simulink library "ddm"  (R2021b)
settings: Solver=VariableStepAuto  StartTime=0.0  StopTime=10.0  RelTol=1e-3
undefined symbols (not defined in the file or in its folder): ENUM_ADASACCSTA_ERROR, ENUM_ADASACCSTA_OFF, ENUM_ADASACCSTA_STANDBY, ENUM_ADASISASTA_OFF, ENUM_ALLOWMOV_ALLOWREADY, ENUM_APS, ENUM_BRKSTA_ERROR, ENUM_BRKSTA_OFF, ENUM_BRKSTA_ON, ENUM_BRKSW_INVALID, ENUM_BRKSW_OFF, ENUM_BRKSW_ON, ENUM_CHGPREACTERRSTA_OBCPRE, ENUM_DCDCFAULTSTA_ANYFAULTLV1, ENUM_DCDCFAULTSTA_ANYFAULTLV2, ENUM_DRIVETRAIN_AWD, ENUM_DRIVETRAIN_FWD, ENUM_DRIVETRAIN_RWD, ENUM_DRSEATSTA_INVALID, ENUM_EDUDRTSTA_NORMAL, ENUM_EPBSTA_APPLIED, ENUM_EPBSTA_RELEASED, ENUM_HVBATTREADYPRE_READY, ENUM_MCUWARN_LV0, ENUM_MCUWARN_LV1, ENUM_MCUWARN_LV2, ENUM_MCUWARN_LV3, ENUM_MCUWARN_NOERROR, ENUM_OBCFAULTSTA_ANYFAULT, ENUM_PAS_R2F2, ENUM_PDFAULT_BATTPDFAIL, ENUM_PDFAULT_DCDCDISABLE, ENUM_PDFAULT_MCUDISABLE, ENUM_PDFAULT_MCUDISCHRG, ENUM_POWERSTA_OFF, ENUM_POWERSTA_ON, ENUM_POWERSTA_READY, ENUM_POWERSTA_STANDBY, ENUM_PRESSINDI_LOW, ENUM_PUFAULT_BATTUPFAIL, ENUM_PUFAULT_DCDCENABLEFAIL, ENUM_PUFAULT_PRECHRGCHKFAIL, ENUM_PUFAULT_SAFETYCHKFAIL, ENUM_PUSTATE_COMPLETED, ENUM_PWRSTASW_OFF, ENUM_PWRSTASW_OFFA, ENUM_PWRSTASW_OFFCHVCHRG, ENUM_PWRSTASW_OFFCLVCHRG, ENUM_PWRSTASW_ON, ENUM_PWRSTASW_ONHVCHRG, ENUM_PWRSTASW_READY, ENUM_PWRSTASW_STANDBY, ENUM_RANGESTA_12IN, ENUM_SHIFTCOMMAND_D, ENUM_SHIFTCOMMAND_N, ENUM_SHIFTCOMMAND_P, ENUM_SHIFTCOMMAND_R, ENUM_VEHMALFUNLV_2ND, ENUM_VEHMALFUNLV_3RD, ENUM_VEHMALFUNLV_4TH ... (+835)
libraries: hcu_lib x750, $bdroot x12, simulink x5
(part 6 of 28)

== system ddm/DDM/DDM/APM/Subsystem8 ==
  USSSta_flg : Inport
  VPMM_SysPwrSta_enum : Inport  Port=2
  VAPM_SNSRLayout_enum : Inport  Port=3
  Constant1 : Constant  Value=ENUM_PWRSTASW_READY
  Constant17 : Constant  Value=ENUM_PWRSTASW_READY
  Constant2 : Constant  Value=ENUM_PWRSTASW_ON
  Constant25 : Constant  Value=FALSE
  Constant3 : Constant  Value=ENUM_PWRSTASW_ON
  Constant5 : Constant  Value=ENUM_APS
  Equal{1..3,5..6} (5 alike) : RelationalOperator  Operator===  OutDataTypeStr=boolean  RndMeth=Simplest
  Logical Operator1 : Logic  Operator=NOT  AllPortsSameDT=off  OutDataTypeStr=boolean
  Logical Operator13 : Logic  Operator=OR  AllPortsSameDT=off  OutDataTypeStr=boolean
  Logical Operator2 : Logic  AllPortsSameDT=off  OutDataTypeStr=boolean
  Logical Operator3 : Logic  Operator=OR  AllPortsSameDT=off  OutDataTypeStr=boolean
  Logical Operator4 : Logic  AllPortsSameDT=off  OutDataTypeStr=boolean
  Switch2 : Switch  Criteria=u2 ~= 0
  Pass_flg : Outport
  CFS_flg : Outport  Port=2
  wires:
  [VPMM_SysPwrSta_enum] -> Equal2/1
  Equal6/1 -> Logical Operator13/1
  Constant17/1 -> Equal2/2
  Constant3/1 -> Equal6/2
  Equal2/1 -> Logical Operator13/2
  [VPMM_SysPwrSta_enum] -> Equal6/1
  Logical Operator13/1 -> Logical Operator2/1
  Logical Operator1/1 -> Logical Operator2/2
  Logical Operator2/1 -> Pass_flg/1
  Logical Operator3/1 -> Logical Operator4/2
  [VPMM_SysPwrSta_enum] -> Equal3/1
  Equal1/1 -> Logical Operator3/2
  Constant2/1 -> Equal3/2
  Constant1/1 -> Equal1/2
  Equal3/1 -> Logical Operator3/1
  [VPMM_SysPwrSta_enum] -> Equal1/1
  Switch2/1 -> Logical Operator4/1, Logical Operator1/1
  Logical Operator4/1 -> CFS_flg/1
  VPMM_SysPwrSta_enum/1 -> [VPMM_SysPwrSta_enum]
  Constant5/1 -> Equal5/2
  VAPM_SNSRLayout_enum/1 -> Equal5/1
  Equal5/1 -> Switch2/2
  Constant25/1 -> Switch2/3
  USSSta_flg/1 -> Switch2/1

== system ddm/DDM/DDM/APM/Subsystem9 ==
  USSSta_flg : Inport
  VPMM_SysPwrSta_enum : Inport  Port=2
  VAPM_SNSRLayout_enum : Inport  Port=3
  Constant1 : Constant  Value=ENUM_PWRSTASW_READY
  Constant17 : Constant  Value=ENUM_PWRSTASW_READY
  Constant2 : Constant  Value=ENUM_PWRSTASW_ON
  Constant25 : Constant  Value=FALSE
  Constant3 : Constant  Value=ENUM_PWRSTASW_ON
  Constant5 : Constant  Value=ENUM_APS
  Equal{1..3,5..6} (5 alike) : RelationalOperator  Operator===  OutDataTypeStr=boolean  RndMeth=Simplest
  Logical Operator1 : Logic  Operator=NOT  AllPortsSameDT=off  OutDataTypeStr=boolean
  Logical Operator13 : Logic  Operator=OR  AllPortsSameDT=off  OutDataTypeStr=boolean
  Logical Operator2 : Logic  AllPortsSameDT=off  OutDataTypeStr=boolean
  Logical Operator3 : Logic  Operator=OR  AllPortsSameDT=off  OutDataTypeStr=boolean
  Logical Operator4 : Logic  AllPortsSameDT=off  OutDataTypeStr=boolean
  Switch2 : Switch  Criteria=u2 ~= 0
  Pass_flg : Outport
  CFS_flg : Outport  Port=2
  wires:
  [VPMM_SysPwrSta_enum] -> Equal2/1
  Equal6/1 -> Logical Operator13/1
  Constant17/1 -> Equal2/2
  Constant3/1 -> Equal6/2
  Equal2/1 -> Logical Operator13/2
  [VPMM_SysPwrSta_enum] -> Equal6/1
  Logical Operator13/1 -> Logical Operator2/1
  Logical Operator1/1 -> Logical Operator2/2
  Logical Operator2/1 -> Pass_flg/1
  Logical Operator3/1 -> Logical Operator4/2
  [VPMM_SysPwrSta_enum] -> Equal3/1
  Equal1/1 -> Logical Operator3/2
  Constant2/1 -> Equal3/2
  Constant1/1 -> Equal1/2
  Equal3/1 -> Logical Operator3/1
  [VPMM_SysPwrSta_enum] -> Equal1/1
  Switch2/1 -> Logical Operator4/1, Logical Operator1/1
  Logical Operator4/1 -> CFS_flg/1
  VPMM_SysPwrSta_enum/1 -> [VPMM_SysPwrSta_enum]
  Constant5/1 -> Equal5/2
  VAPM_SNSRLayout_enum/1 -> Equal5/1
  Equal5/1 -> Switch2/2
  Constant25/1 -> Switch2/3
  USSSta_flg/1 -> Switch2/1

== system ddm/DDM/DDM/PMM/Brake switch signal abnormal ==
  task_time_s : Inport
  VPMM_PwrStaSW_enum : Inport  Port=2
  VPMM_PowerSta_enum : Inport  Port=3
  VINP_BrakeSWGPIO_flg : Inport  Port=4
  VINP_BrakeLampSW_flg : Inport  Port=5
  VDDM_ESC5NoComCFS_flg : Inport  Port=6
  VDDM_ESC5RCErrCFS_flg : Inport  Port=7
  VDDM_ESC5CSErrCFS_flg : Inport  Port=8
  VINP_DrStdAErrSta_enum : Inport  Port=9
  VINP_BrkSWSta_flg : Inport  Port=10
  VDDM_ESC7NoComCFS_flg : Inport  Port=11
  VDDM_ESC7RCErrCFS_flg : Inport  Port=12
  VDDM_ESC7CSErrCFS_flg : Inport  Port=13
  VINP_BrkPedalPosSta_enum : Inport  Port=14
  VINP_BrkPedalPos_pct : Inport  Port=15
  DTC_clear_request : Inport  Port=16
  Brake switch signal abnormal : Subsystem
  Brake switch signal abnormal and no backup signal : Subsystem
  Constant : Constant  Value=TRUE
  Constant1 : Constant  Value=ENUM_BRKSTA_ERROR
  Constant2 : Constant  Value=ENUM_BRKSTA_ON
  Constant3 : Constant  Value=ENUM_BRKSTA_OFF
  Constant4 : Constant  Value=FALSE
  Constant5 : Constant  Value=ENUM_BRKSTA_ERROR
  Constant6 : Constant  Value=ENUM_BRKSTA_ON
  Constant7 : Constant  Value=ENUM_BRKSTA_OFF
  Constant8 : Constant  Value=KDDM_BrkPedalPos_pct
  Equal : RelationalOperator  Operator===  OutDataTypeStr=boolean  RndMeth=Simplest
  Equal1 : RelationalOperator  Operator===  OutDataTypeStr=boolean  RndMeth=Simplest
  Equal2 : RelationalOperator  OutDataTypeStr=boolean  RndMeth=Simplest
  Logical Operator : Logic  Operator=OR  Inputs=4  AllPortsSameDT=off  OutDataTypeStr=boolean
  Logical Operator1 : Logic  Operator=OR  Inputs=4  AllPortsSameDT=off  OutDataTypeStr=boolean
  Subsystem : Subsystem
  Switch{,1..3} (4 alike) : Switch  Criteria=u2 > Threshold
  VDDM_BrkSWErrDTC_raw32 : Outport
  VDDM_BrkSWNoBacDTC_raw32 : Outport  Port=2
  VDDM_BrakeSW_enum : Outport  Port=3
  VDDM_CANBrkSW2Sta_enum : Outport  Port=4
  VDDM_BrkPedalPosSta_enum : Outport  Port=5
  VDDM_EDriveSysErrBrake_flg : Outport  Port=6
  VDDM_VCUBrkSWSta_enum : Outport  Port=7
  wires:
  [VDDM_BrakeSW_enum] -> Brake switch signal abnormal and no backup signal/7(VDDM_BrakeSW_enum)
  [VDDM_BrkSWPass_flg] -> Brake switch signal abnormal and no backup signal/5(BrkSWPass)
  [VDDM_BrkSWNoBac_flg] -> Brake switch signal abnormal and no backup signal/4(BrkSWNoBac)
  [VDDM_BrkSWPass_flg] -> Brake switch signal abnormal/5(BrkSWPass)
  [VDDM_BrkSWErr_flg] -> Brake switch signal abnormal/4(BrkSWErr)
  Subsystem/3(BrkSWPass) -> [VDDM_BrkSWPass_flg]  "VDDM_BrkSWPass_flg"
  Subsystem/2(BrkSWNoBac) -> [VDDM_BrkSWNoBac_flg]  "VDDM_BrkSWNoBac_flg"
  Subsystem/4(VDDM_BrakeSW_enum) -> [VDDM_BrakeSW_enum]  "VDDM_BrakeSW_enum"
  Subsystem/1(BrkSWErr) -> [VDDM_BrkSWErr_flg]  "VDDM_BrkSWErr_flg"
  VINP_BrakeLampSW_flg/1 -> Subsystem/3(Brake_Stop_Lamp)
  VINP_BrakeSWGPIO_flg/1 -> Subsystem/2(BrakeSW)
  [VDDM_BrkPedalPosSta_enum] -> Subsystem/4(BrkPedalPos_enum)
  [VDDM_CANBrkSW2Sta_enum] -> Subsystem/1(VDDM_CANBSW2S_enum)
  [DTC_clear_request] -> Brake switch signal abnormal and no backup signal/6(DTC_clear_request)
  [DTC_clear_request] -> Brake switch signal abnormal/6(DTC_clear_request)
  DTC_clear_request/1 -> [DTC_clear_request]
  Brake switch signal abnormal and no backup signal/2(VDDM_VCUBrkSWSta_enum) -> VDDM_VCUBrkSWSta_enum/1
  Brake switch signal abnormal/2(VDDM_EDriveSysErrBrake_flg) -> VDDM_EDriveSysErrBrake_flg/1
  [VDDM_BrakeSW_enum] -> VDDM_BrakeSW_enum/1
  [VDDM_CANBrkSW2Sta_enum] -> VDDM_CANBrkSW2Sta_enum/1
  [VDDM_BrkPedalPosSta_enum] -> VDDM_BrkPedalPosSta_enum/1
  Switch2/1 -> [VDDM_BrkPedalPosSta_enum]  "VDDM_BrkPedalPosSta_enum"
  Switch/1 -> [VDDM_CANBrkSW2Sta_enum]  "VDDM_CANBrkSW2Sta_enum"
  Brake switch signal abnormal and no backup signal/1(VDDM_BrkSWNoBacDTC_raw32) -> VDDM_BrkSWNoBacDTC_raw32/1
  Brake switch signal abnormal/1(VDDM_BrkSWErrDTC_raw32) -> VDDM_BrkSWErrDTC_raw32/1
  Equal2/1 -> Switch3/2
  Constant8/1 -> Equal2/2
  VINP_BrkPedalPos_pct/1 -> Equal2/1
  VINP_BrkPedalPosSta_enum/1 -> Equal1/1
  Constant4/1 -> Equal1/2
  VDDM_ESC7CSErrCFS_flg/1 -> Logical Operator1/3
  VDDM_ESC7RCErrCFS_flg/1 -> Logical Operator1/2
  VDDM_ESC7NoComCFS_flg/1 -> Logical Operator1/1
  Equal1/1 -> Logical Operator1/4
  Switch3/1 -> Switch2/3
  Logical Operator1/1 -> Switch2/2
  Constant5/1 -> Switch2/1
  Constant6/1 -> Switch3/1
  Constant7/1 -> Switch3/3
  Constant3/1 -> Switch1/3
  Constant2/1 -> Switch1/1
  VINP_BrkSWSta_flg/1 -> Switch1/2
  Constant1/1 -> Switch/1
  Logical Operator/1 -> Switch/2
  Switch1/1 -> Switch/3
  Equal/1 -> Logical Operator/4
  VDDM_ESC5NoComCFS_flg/1 -> Logical Operator/1
  VDDM_ESC5RCErrCFS_flg/1 -> Logical Operator/2
  VDDM_ESC5CSErrCFS_flg/1 -> Logical Operator/3
  Constant/1 -> Equal/2
  VINP_DrStdAErrSta_enum/1 -> Equal/1
  task_time_s/1 -> [task_time_s]
  VPMM_PwrStaSW_enum/1 -> [VPMM_PwrStaSW_enum]
  VPMM_PowerSta_enum/1 -> [VPMM_PowerSta_enum]
  [task_time_s] -> Brake switch signal abnormal/1(task_time_s)
  [VPMM_PwrStaSW_enum] -> Brake switch signal abnormal/3(VPMM_PwrStaSW_enum)
  [VPMM_PowerSta_enum] -> Brake switch signal abnormal/2(VPMM_PowerSta_enum)
  [task_time_s] -> Brake switch signal abnormal and no backup signal/1(task_time_s)
  [VPMM_PowerSta_enum] -> Brake switch signal abnormal and no backup signal/2(VPMM_PowerSta_enum)
  [VPMM_PwrStaSW_enum] -> Brake switch signal abnormal and no backup signal/3(VPMM_PwrStaSW_enum)

== system ddm/DDM/DDM/PMM/Comm err ==
  note: CAN1 EPAS2
  note: CAN3 BMS6
  note: CAN3 BMS1
  note: CAN3 CCU1
  note: CAN3 CCU2
  note: CAN1 ABM1
  task_time_s : Inport
  VPMM_PowerSta_enum : Inport  Port=2
  VPMM_PwrStaSW_enum : Inport  Port=3
  VDDM_C3BMS6RCChk_flg : Inport  Port=4
  VDDM_C3BMS6CSChk_flg : Inport  Port=5
  VDDM_C3BMS6LCChk_flg : Inport  Port=6
  VDDM_C3BMS1RCChk_flg : Inport  Port=7
  VDDM_C3BMS1CSChk_flg : Inport  Port=8
  VDDM_C3BMS1LCChk_flg : Inport  Port=9
  VDDM_C3CCU1RCChk_flg : Inport  Port=10
  VDDM_C3CCU1CSChk_flg : Inport  Port=11
  VDDM_C3CCU1LCChk_flg : Inport  Port=12
  VDDM_C3CCU2RCChk_flg : Inport  Port=13
  VDDM_C3CCU2CSChk_flg : Inport  Port=14
  VDDM_C3CCU2LCChk_flg : Inport  Port=15
  VDDM_C1ABM1RCChk_flg : Inport  Port=16
  VDDM_C1ABM1CSChk_flg : Inport  Port=17
  VDDM_C1ABM1LCChk_flg : Inport  Port=18
  No_CAN3_BUS_OFF : Inport  Port=19
  No_CAN1_BUS_OFF : Inport  Port=20
  DTC_clear_request : Inport  Port=21
  VDDM_C1EPAS2LCChk_flg : Inport  Port=22
  FDC lost communication with EPAS2 : Subsystem
  OR : Logic  Operator=OR  Inputs=3  AllPortsSameDT=off  OutDataTypeStr=boolean
  The CAN signal between VCU and ABM1 is discontinuous : Subsystem
  The CAN signal between VCU and ABM1 is incomplete : Subsystem
  The CAN signal between VCU and BMS1 is discontinuous : Subsystem
  The CAN signal between VCU and BMS1 is incomplete : Subsystem
  The CAN signal between VCU and BMS6 is discontinuous : Subsystem
  The CAN signal between VCU and BMS6 is incomplete : Subsystem
  The CAN signal between VCU and CCU1 is discontinuous : Subsystem
  The CAN signal between VCU and CCU1 is incomplete : Subsystem
  The CAN signal between VCU and CCU2 is discontinuous : Subsystem
  The CAN signal between VCU and CCU2 is incomplete : Subsystem
  VCU lost communication with ABM1 : Subsystem
  VCU lost communication with BMS1 : Subsystem
  VCU lost communication with BMS6 : Subsystem
  VCU lost communication with CCU1 : Subsystem
  VCU lost communication with CCU2 : Subsystem
  VDDM_C3BMS6RCDTC_raw32 : Outport
  VDDM_C3BMS6CSDTC_raw32 : Outport  Port=2
  VDDM_C3BMS6LCDTC_raw32 : Outport  Port=3
  VDDM_C3BMS1RCDTC_raw32 : Outport  Port=4
  VDDM_C3BMS1CSDTC_raw32 : Outport  Port=5
  VDDM_C3BMS1LCDTC_raw32 : Outport  Port=6
  VDDM_C3CCU1RCDTC_raw32 : Outport  Port=7
  VDDM_C3CCU1CSDTC_raw32 : Outport  Port=8
  VDDM_C3CCU1LCDTC_raw32 : Outport  Port=9
  VDDM_C3CCU2RCDTC_raw32 : Outport  Port=10
  VDDM_C3CCU2CSDTC_raw32 : Outport  Port=11
  VDDM_C3CCU2LCDTC_raw32 : Outport  Port=12
  VDDM_C1ABM1RCDTC_raw32 : Outport  Port=13
  VDDM_C1ABM1CSDTC_raw32 : Outport  Port=14
  VDDM_C1ABM1LCDTC_raw32 : Outport  Port=15
  VDDM_EDriveSysErrABMCAN_flg : Outport  Port=16
  VDDM_C3BMS6CSCFS_flg : Outport  Port=17
  VDDM_C3BMS6RCCFS_flg : Outport  Port=18
  VDDM_C3BMS6LCCFS_flg : Outport  Port=19
  VDDM_C3CCU2CSCFS_flg : Outport  Port=20
  VDDM_C3CCU2LCCFS_flg : Outport  Port=21
  VDDM_C3CCU2RCCFS_flg : Outport  Port=22
  VDDM_C1EPAS2LCDTC_raw32 : Outport  Port=23
  wires:
  [task_time_s] -> FDC lost communication with EPAS2/1(task_time_s)
  FDC lost communication with EPAS2/2(VDDM_C1EPAS2LCCFS_flg) -> [VDDM_C1EPAS2LCCFS_flg]
  [VPMM_PowerSta_enum] -> FDC lost communication with EPAS2/2(VPMM_PowerSta_enum)
  [VPMM_PwrStaSW_enum] -> FDC lost communication with EPAS2/3(VPMM_PwrStaSW_enum)
  VDDM_C1EPAS2LCChk_flg/1 -> FDC lost communication with EPAS2/4(VDDM_C1EPAS2LCChk_flg)
  [No_CAN1_BUS_OFF] -> FDC lost communication with EPAS2/5(No_CAN1_BUS_OFF)
  [DTC_clear_request] -> FDC lost communication with EPAS2/6(DTC_clear_request)
  FDC lost communication with EPAS2/1(VDDM_C1EPAS2LCDTC_raw32) -> VDDM_C1EPAS2LCDTC_raw32/1
  The CAN signal between VCU and CCU2 is discontinuous/2(VDDM_C3CCU2RCCFS_flg) -> VDDM_C3CCU2RCCFS_flg/1
  [VDDM_C3CCU2LCCFS_flg] -> VDDM_C3CCU2LCCFS_flg/1
  The CAN signal between VCU and CCU2 is incomplete/2(VDDM_C3CCU2CSCFS_flg) -> VDDM_C3CCU2CSCFS_flg/1
  The CAN signal between VCU and BMS6 is discontinuous/2(VDDM_C3BMS6RCCFS_flg) -> VDDM_C3BMS6RCCFS_flg/1
  [VDDM_C3BMS6LCCFS_flg] -> VDDM_C3BMS6LCCFS_flg/1
  The CAN signal between VCU and BMS6 is incomplete/2(VDDM_C3BMS6CSCFS_flg) -> VDDM_C3BMS6CSCFS_flg/1
  The CAN signal between VCU and CCU1 is discontinuous/1(VDDM_C3CCU1RCDTC_raw32) -> VDDM_C3CCU1RCDTC_raw32/1
  VCU lost communication with BMS6/1(VDDM_C3BMS6LCDTC_raw32) -> VDDM_C3BMS6LCDTC_raw32/1
  VCU lost communication with ABM1/1(VDDM_C1ABM1LCDTC_raw32) -> VDDM_C1ABM1LCDTC_raw32/1
  The CAN signal between VCU and ABM1 is incomplete/1(VDDM_C1ABM1CSDTC_raw32) -> VDDM_C1ABM1CSDTC_raw32/1
  The CAN signal between VCU and ABM1 is discontinuous/1(VDDM_C1ABM1RCDTC_raw32) -> VDDM_C1ABM1RCDTC_raw32/1
  VCU lost communication with CCU2/1(VDDM_C3CCU2LCDTC_raw32) -> VDDM_C3CCU2LCDTC_raw32/1
  The CAN signal between VCU and CCU2 is incomplete/1(VDDM_C3CCU2CSDTC_raw32) -> VDDM_C3CCU2CSDTC_raw32/1
  The CAN signal between VCU and CCU2 is discontinuous/1(VDDM_C3CCU2RCDTC_raw32) -> VDDM_C3CCU2RCDTC_raw32/1
  VCU lost communication with CCU1/1(VDDM_C3CCU1LCDTC_raw32) -> VDDM_C3CCU1LCDTC_raw32/1
  The CAN signal between VCU and CCU1 is incomplete/1(VDDM_C3CCU1CSDTC_raw32) -> VDDM_C3CCU1CSDTC_raw32/1
  VCU lost communication with BMS1/1(VDDM_C3BMS1LCDTC_raw32) -> VDDM_C3BMS1LCDTC_raw32/1
  The CAN signal between VCU and BMS1 is incomplete/1(VDDM_C3BMS1CSDTC_raw32) -> VDDM_C3BMS1CSDTC_raw32/1
  The CAN signal between VCU and BMS1 is discontinuous/1(VDDM_C3BMS1RCDTC_raw32) -> VDDM_C3BMS1RCDTC_raw32/1
  The CAN signal between VCU and BMS6 is incomplete/1(VDDM_C3BMS6CSDTC_raw32) -> VDDM_C3BMS6CSDTC_raw32/1
  The CAN signal between VCU and BMS6 is discontinuous/1(VDDM_C3BMS6RCDTC_raw32) -> VDDM_C3BMS6RCDTC_raw32/1
  DTC_clear_request/1 -> [DTC_clear_request]
  No_CAN1_BUS_OFF/1 -> [No_CAN1_BUS_OFF]
  No_CAN3_BUS_OFF/1 -> [No_CAN3_BUS_OFF]
  OR/1 -> VDDM_EDriveSysErrABMCAN_flg/1
  [VDDM_EDriveSysErrABMLC_flg] -> OR/3
  [VDDM_EDriveSysErrABMRC_flg] -> OR/1
  [VDDM_EDriveSysErrABMCS_flg] -> OR/2
  VCU lost communication with ABM1/3(LC_EDriveSysErr_VCUErr_flg) -> [VDDM_EDriveSysErrABMLC_flg]
  [DTC_clear_request] -> VCU lost communication with ABM1/6(DTC_clear_request)
  [No_CAN1_BUS_OFF] -> VCU lost communication with ABM1/5(No_CAN1_BUS_OFF)
  The CAN signal between VCU and ABM1 is incomplete/2(CS_EDriveSysErr_VCUErr_flg) -> [VDDM_EDriveSysErrABMCS_flg]
  The CAN signal between VCU and ABM1 is discontinuous/2(RC_EDriveSysErr_VCUErr_flg) -> [VDDM_EDriveSysErrABMRC_flg]
  [DTC_clear_request] -> The CAN signal between VCU and ABM1 is incomplete/7(DTC_clear_request)
  [No_CAN1_BUS_OFF] -> The CAN signal between VCU and ABM1 is incomplete/6(No_CAN1_BUS_OFF)
  [DTC_clear_request] -> The CAN signal between VCU and ABM1 is discontinuous/7(DTC_clear_request)
  [No_CAN1_BUS_OFF] -> The CAN signal between VCU and ABM1 is discontinuous/6(No_CAN1_BUS_OFF)
  [DTC_clear_request] -> VCU lost communication with CCU2/6(DTC_clear_request)
  [No_CAN3_BUS_OFF] -> VCU lost communication with CCU2/5(No_CAN3_BUS_OFF)
  [DTC_clear_request] -> The CAN signal between VCU and CCU2 is incomplete/7(DTC_clear_request)
  [No_CAN3_BUS_OFF] -> The CAN signal between VCU and CCU2 is incomplete/6(No_CAN3_BUS_OFF)
  [DTC_clear_request] -> The CAN signal between VCU and CCU2 is discontinuous/7(DTC_clear_request)
  [No_CAN3_BUS_OFF] -> The CAN signal between VCU and CCU2 is discontinuous/6(No_CAN3_BUS_OFF)
  [DTC_clear_request] -> VCU lost communication with CCU1/6(DTC_clear_request)
  [No_CAN3_BUS_OFF] -> VCU lost communication with CCU1/5(No_CAN3_BUS_OFF)
  [DTC_clear_request] -> The CAN signal between VCU and CCU1 is incomplete/7(DTC_clear_request)
  [No_CAN3_BUS_OFF] -> The CAN signal between VCU and CCU1 is incomplete/6(No_CAN3_BUS_OFF)
  [DTC_clear_request] -> The CAN signal between VCU and CCU1 is discontinuous/7(DTC_clear_request)
  [No_CAN3_BUS_OFF] -> The CAN signal between VCU and CCU1 is discontinuous/6(No_CAN3_BUS_OFF)
  [DTC_clear_request] -> VCU lost communication with BMS1/6(DTC_clear_request)
  [No_CAN3_BUS_OFF] -> VCU lost communication with BMS1/5(No_CAN3_BUS_OFF)
  [DTC_clear_request] -> The CAN signal between VCU and BMS1 is incomplete/7(DTC_clear_request)
  [No_CAN3_BUS_OFF] -> The CAN signal between VCU and BMS1 is incomplete/6(No_CAN3_BUS_OFF)
  [VDDM_C3BMS1LCCFS_flg] -> The CAN signal between VCU and BMS1 is discontinuous/5(VDDM_C3BMS1LCCFS_flg)
  [DTC_clear_request] -> The CAN signal between VCU and BMS1 is discontinuous/7(DTC_clear_request)
  [DTC_clear_request] -> VCU lost communication with BMS6/6(DTC_clear_request)
  [No_CAN3_BUS_OFF] -> VCU lost communication with BMS6/5(No_CAN3_BUS_OFF)
  [VDDM_C3BMS6LCCFS_flg] -> The CAN signal between VCU and BMS6 is incomplete/5(VDDM_C3BMS6LCCFS_flg)
  [VDDM_C3BMS6LCCFS_flg] -> The CAN signal between VCU and BMS6 is discontinuous/5(VDDM_C3BMS6LCCFS_flg)
  [DTC_clear_request] -> The CAN signal between VCU and BMS6 is incomplete/7(DTC_clear_request)
  [DTC_clear_request] -> The CAN signal between VCU and BMS6 is discontinuous/7(DTC_clear_request)
  VDDM_C3BMS6LCChk_flg/1 -> VCU lost communication with BMS6/4(VDDM_C3BMS6LCChk_flg)
  VDDM_C3BMS6CSChk_flg/1 -> The CAN signal between VCU and BMS6 is incomplete/4(VDDM_C3BMS6CSChk_flg)
  VDDM_C3BMS6RCChk_flg/1 -> The CAN signal between VCU and BMS6 is discontinuous/4(VDDM_C3BMS6RCChk_flg)
  task_time_s/1 -> [task_time_s]
  VPMM_PwrStaSW_enum/1 -> [VPMM_PwrStaSW_enum]
  VPMM_PowerSta_enum/1 -> [VPMM_PowerSta_enum]
  VDDM_C3CCU2RCChk_flg/1 -> The CAN signal between VCU and CCU2 is discontinuous/4(VDDM_C3CCU2RCChk_flg)
  VDDM_C3CCU2LCChk_flg/1 -> VCU lost communication with CCU2/4(VDDM_C3CCU2LCChk_flg)
  VDDM_C3CCU1CSChk_flg/1 -> The CAN signal between VCU and CCU1 is incomplete/4(VDDM_C3CCU1CSChk_flg)
  VDDM_C3BMS1CSChk_flg/1 -> The CAN signal between VCU and BMS1 is incomplete/4(VDDM_C3BMS1CSChk_flg)
  VDDM_C1ABM1CSChk_flg/1 -> The CAN signal between VCU and ABM1 is incomplete/4(VDDM_C1ABM1CSChk_flg)
  VDDM_C1ABM1RCChk_flg/1 -> The CAN signal between VCU and ABM1 is discontinuous/4(VDDM_C1ABM1RCChk_flg)
  VDDM_C3CCU1RCChk_flg/1 -> The CAN signal between VCU and CCU1 is discontinuous/4(VDDM_C3CCU1RCChk_flg)
  VDDM_C3CCU1LCChk_flg/1 -> VCU lost communication with CCU1/4(VDDM_C3CCU1LCChk_flg)
  VDDM_C3BMS1RCChk_flg/1 -> The CAN signal between VCU and BMS1 is discontinuous/4(VDDM_C3BMS1RCChk_flg)
  VDDM_C3CCU2CSChk_flg/1 -> The CAN signal between VCU and CCU2 is incomplete/4(VDDM_C3CCU2CSChk_flg)
  [VPMM_PowerSta_enum] -> The CAN signal between VCU and ABM1 is discontinuous/2(VPMM_PowerSta_enum)
  [task_time_s] -> The CAN signal between VCU and ABM1 is discontinuous/1(task_time_s)
  [VDDM_C1ABM1LCCFS_flg] -> The CAN signal between VCU and ABM1 is incomplete/5(VDDM_C1ABM1LCCFS_flg)
  [VPMM_PwrStaSW_enum] -> The CAN signal between VCU and CCU2 is incomplete/3(VPMM_PwrStaSW_enum)
  [VPMM_PowerSta_enum] -> The CAN signal between VCU and ABM1 is incomplete/2(VPMM_PowerSta_enum)
  [VPMM_PowerSta_enum] -> VCU lost communication with CCU2/2(VPMM_PowerSta_enum)
  [task_time_s] -> The CAN signal between VCU and CCU2 is incomplete/1(task_time_s)
  [VPMM_PwrStaSW_enum] -> The CAN signal between VCU and CCU2 is discontinuous/3(VPMM_PwrStaSW_enum)
  VCU lost communication with BMS6/2(VDDM_C3BMS6LCCFS_flg) -> [VDDM_C3BMS6LCCFS_flg]
  [VPMM_PowerSta_enum] -> The CAN signal between VCU and CCU1 is discontinuous/2(VPMM_PowerSta_enum)
  [VDDM_C3CCU1LCCFS_flg] -> The CAN signal between VCU and CCU1 is incomplete/5(VDDM_C3CCU1LCCFS_flg)
  [VPMM_PwrStaSW_enum] -> VCU lost communication with CCU1/3(VPMM_PwrStaSW_enum)
  [VPMM_PowerSta_enum] -> VCU lost communication with CCU1/2(VPMM_PowerSta_enum)
  [VPMM_PwrStaSW_enum] -> The CAN signal between VCU and CCU1 is incomplete/3(VPMM_PwrStaSW_enum)
  [VPMM_PwrStaSW_enum] -> The CAN signal between VCU and CCU1 is discontinuous/3(VPMM_PwrStaSW_enum)
  [VPMM_PwrStaSW_enum] -> The CAN signal between VCU and BMS6 is discontinuous/3(VPMM_PwrStaSW_enum)
  [task_time_s] -> The CAN signal between VCU and CCU1 is discontinuous/1(task_time_s)
  [VPMM_PowerSta_enum] -> The CAN signal between VCU and CCU1 is incomplete/2(VPMM_PowerSta_enum)
  [No_CAN3_BUS_OFF] -> The CAN signal between VCU and BMS6 is discontinuous/6(No_CAN3_BUS_OFF)
  VCU lost communication with CCU1/2(VDDM_C3CCU1LCCFS_flg) -> [VDDM_C3CCU1LCCFS_flg]
  [No_CAN3_BUS_OFF] -> The CAN signal between VCU and BMS1 is discontinuous/6(No_CAN3_BUS_OFF)
  [task_time_s] -> VCU lost communication with BMS1/1(task_time_s)
  [VPMM_PowerSta_enum] -> VCU lost communication with BMS6/2(VPMM_PowerSta_enum)
  [VPMM_PwrStaSW_enum] -> The CAN signal between VCU and BMS1 is incomplete/3(VPMM_PwrStaSW_enum)
  [VPMM_PowerSta_enum] -> The CAN signal between VCU and CCU2 is incomplete/2(VPMM_PowerSta_enum)
  [task_time_s] -> VCU lost communication with CCU1/1(task_time_s)
  [VDDM_C3BMS1LCCFS_flg] -> The CAN signal between VCU and BMS1 is incomplete/5(VDDM_C3BMS1LCCFS_flg)
  [VPMM_PowerSta_enum] -> The CAN signal between VCU and BMS1 is incomplete/2(VPMM_PowerSta_enum)
  VDDM_C3BMS1LCChk_flg/1 -> VCU lost communication with BMS1/4(VDDM_C3BMS1LCChk_flg)
  [task_time_s] -> The CAN signal between VCU and ABM1 is incomplete/1(task_time_s)
  [VPMM_PowerSta_enum] -> The CAN signal between VCU and BMS1 is discontinuous/2(VPMM_PowerSta_enum)
  [No_CAN3_BUS_OFF] -> The CAN signal between VCU and BMS6 is incomplete/6(No_CAN3_BUS_OFF)
  [VPMM_PwrStaSW_enum] -> VCU lost communication with BMS1/3(VPMM_PwrStaSW_enum)
  [VDDM_C3CCU2LCCFS_flg] -> The CAN signal between VCU and CCU2 is discontinuous/5(VDDM_C3CCU2LCCFS_flg)
  [VPMM_PowerSta_enum] -> The CAN signal between VCU and BMS6 is incomplete/2(VPMM_PowerSta_enum)
  [VDDM_C3CCU1LCCFS_flg] -> The CAN signal between VCU and CCU1 is discontinuous/5(VDDM_C3CCU1LCCFS_flg)
  [VPMM_PwrStaSW_enum] -> The CAN signal between VCU and BMS1 is discontinuous/3(VPMM_PwrStaSW_enum)
  [task_time_s] -> The CAN signal between VCU and BMS1 is discontinuous/1(task_time_s)
  [VPMM_PowerSta_enum] -> VCU lost communication with BMS1/2(VPMM_PowerSta_enum)
  [VPMM_PowerSta_enum] -> The CAN signal between VCU and CCU2 is discontinuous/2(VPMM_PowerSta_enum)
  VCU lost communication with BMS1/2(VDDM_C3BMS1LCCFS_flg) -> [VDDM_C3BMS1LCCFS_flg]
  [task_time_s] -> The CAN signal between VCU and CCU1 is incomplete/1(task_time_s)
  [VDDM_C1ABM1LCCFS_flg] -> The CAN signal between VCU and ABM1 is discontinuous/5(VDDM_C1ABM1LCCFS_flg)
  [task_time_s] -> The CAN signal between VCU and BMS6 is incomplete/1(task_time_s)
  VDDM_C1ABM1LCChk_flg/1 -> VCU lost communication with ABM1/4(VDDM_C1ABM1LCChk_flg)
  [VPMM_PwrStaSW_enum] -> The CAN signal between VCU and ABM1 is incomplete/3(VPMM_PwrStaSW_enum)
  VCU lost communication with ABM1/2(VDDM_C1ABM1LCCFS_flg) -> [VDDM_C1ABM1LCCFS_flg]
  [task_time_s] -> VCU lost communication with CCU2/1(task_time_s)
  [VPMM_PowerSta_enum] -> The CAN signal between VCU and BMS6 is discontinuous/2(VPMM_PowerSta_enum)
  [VPMM_PwrStaSW_enum] -> The CAN signal between VCU and ABM1 is discontinuous/3(VPMM_PwrStaSW_enum)
  [VPMM_PowerSta_enum] -> VCU lost communication with ABM1/2(VPMM_PowerSta_enum)
  [VPMM_PwrStaSW_enum] -> VCU lost communication with BMS6/3(VPMM_PwrStaSW_enum)
  [task_time_s] -> The CAN signal between VCU and BMS1 is incomplete/1(task_time_s)
  [task_time_s] -> VCU lost communication with ABM1/1(task_time_s)
  VCU lost communication with CCU2/2(VDDM_C3CCU2LCCFS_flg) -> [VDDM_C3CCU2LCCFS_flg]
  [VPMM_PwrStaSW_enum] -> VCU lost communication with ABM1/3(VPMM_PwrStaSW_enum)
  [task_time_s] -> The CAN signal between VCU and BMS6 is discontinuous/1(task_time_s)
  [task_time_s] -> The CAN signal between VCU and CCU2 is discontinuous/1(task_time_s)
  [task_time_s] -> VCU lost communication with BMS6/1(task_time_s)
  [VPMM_PwrStaSW_enum] -> VCU lost communication with CCU2/3(VPMM_PwrStaSW_enum)
  [VPMM_PwrStaSW_enum] -> The CAN signal between VCU and BMS6 is incomplete/3(VPMM_PwrStaSW_enum)
  [VDDM_C3CCU2LCCFS_flg] -> The CAN signal between VCU and CCU2 is incomplete/5(VDDM_C3CCU2LCCFS_flg)

== system ddm/DDM/DDM/PMM/Fault level ==
  task_time_s : Inport
  VPMM_PwrStaSW_enum : Inport  Port=2
  VPMM_PowerSta_enum : Inport  Port=3
  VINP_BMSWarn1_flg : Inport  Port=4
  VINP_BMSWarn2_flg : Inport  Port=5
  VINP_BMSWarn3_flg : Inport  Port=6
  VINP_BMSWarn4_flg : Inport  Port=7
  VINP_BMSWarn5_flg : Inport  Port=8
  VINP_BMSWarn6_flg : Inport  Port=9
  VINP_BMSWarn7_flg : Inport  Port=10
  VINP_BMSWarn8_flg : Inport  Port=11
  VINP_DCDCFaultSta_enum : Inport  Port=12
  VPMM_DrivetrainSelect_enum : Inport  Port=13
  VDDM_C3BMS6LCCFS_flg : Inport  Port=14
  VDDM_C3CCU2LCCFS_flg : Inport  Port=15
  VDDM_MCUF1NoComCFS_flg : Inport  Port=16
  VDDM_MCUR1NoComCFS_flg : Inport  Port=17
  VINP_MCUWarnF_enum : Inport  Port=18
  VINP_MCUWarnR_enum : Inport  Port=19
  VINP_OBCFaultSta_enum : Inport  Port=20
  DTC_clear_request : Inport  Port=21
  No_CAN3_BUS_OFF : Inport  Port=22
  Fault level 1 subsystem error : Subsystem
  Fault level 2 subsystem error : Subsystem
  Fault level 3 subsystem error : Subsystem
  Fault level 4 subsystem error : Subsystem
  VDDM_Lv1ErrDTC_raw32 : Outport
  VDDM_Lv2ErrCFS_flg : Outport  Port=2
  VDDM_Lv3ErrDTC_raw32 : Outport  Port=3
  VDDM_Lv4ErrDTC_raw32 : Outport  Port=4
  wires:
  [No_CAN3_BUS_OFF] -> Fault level 4 subsystem error/8(No_CAN3_BUS_OFF)
  [DTC_clear_request] -> Fault level 4 subsystem error/7(DTC_clear_request)
  [DTC_clear_request] -> Fault level 3 subsystem error/11(DTC_clear_request)
  [No_CAN3_BUS_OFF] -> Fault level 3 subsystem error/12(No_CAN3_BUS_OFF)
  [No_CAN3_BUS_OFF] -> Fault level 2 subsystem error/15(No_CAN3_BUS_OFF)
  [DTC_clear_request] -> Fault level 2 subsystem error/14(DTC_clear_request)
  [DTC_clear_request] -> Fault level 1 subsystem error/16(DTC_clear_request)
  [No_CAN3_BUS_OFF] -> Fault level 1 subsystem error/17(No_CAN3_BUS_OFF)
  DTC_clear_request/1 -> [DTC_clear_request]
  No_CAN3_BUS_OFF/1 -> [No_CAN3_BUS_OFF]
  [VINP_MCUWarnR_enum] -> Fault level 1 subsystem error/13(VINP_MCUWarnR_enum)
  [VINP_MCUWarnF_enum] -> Fault level 1 subsystem error/12(VINP_MCUWarnF_enum)
  Fault level 4 subsystem error/1(VDDM_Lv4ErrDTC_raw32) -> VDDM_Lv4ErrDTC_raw32/1
  Fault level 3 subsystem error/1(VDDM_Lv3ErrDTC_raw32) -> VDDM_Lv3ErrDTC_raw32/1
  Fault level 2 subsystem error/1(VDDM_Lv2ErrDTC_raw32) -> VDDM_Lv2ErrCFS_flg/1
  Fault level 1 subsystem error/1(VDDM_Lv1ErrDTC_raw32) -> VDDM_Lv1ErrDTC_raw32/1
  [VINP_MCUWarnF_enum] -> Fault level 3 subsystem error/8(VINP_MCUWarnF_enum)
  [VINP_MCUWarnR_enum] -> Fault level 3 subsystem error/9(VINP_MCUWarnR_enum)
  [VPMM_DrivetrainSelect_enum] -> Fault level 3 subsystem error/10(VPMM_DrivetrainSelect_enum)
  [VINP_MCUWarnR_enum] -> Fault level 2 subsystem error/12(VINP_MCUWarnR_enum)
  [VINP_MCUWarnF_enum] -> Fault level 2 subsystem error/11(VINP_MCUWarnF_enum)
  [VPMM_DrivetrainSelect_enum] -> Fault level 2 subsystem error/13(VPMM_DrivetrainSelect_enum)
  [VINP_OBCFaultSta_enum] -> Fault level 1 subsystem error/14(VINP_OBCFaultSta_enum)
  VINP_OBCFaultSta_enum/1 -> [VINP_OBCFaultSta_enum]
  VINP_MCUWarnR_enum/1 -> [VINP_MCUWarnR_enum]
  VINP_MCUWarnF_enum/1 -> [VINP_MCUWarnF_enum]
  VINP_BMSWarn3_flg/1 -> Fault level 1 subsystem error/10(VINP_BMSWarn3_flg)
  VINP_BMSWarn2_flg/1 -> Fault level 1 subsystem error/9(VINP_BMSWarn2_flg)
  VINP_BMSWarn1_flg/1 -> Fault level 1 subsystem error/8(VINP_BMSWarn1_flg)
  [VDDM_C3CCU2LCCFS_flg] -> Fault level 2 subsystem error/5(VDDM_C3CCU2LCCFS_flg)
  [VDDM_C3CCU2LCCFS_flg] -> Fault level 1 subsystem error/5(VDDM_C3CCU2LCCFS_flg)
  VDDM_C3CCU2LCCFS_flg/1 -> [VDDM_C3CCU2LCCFS_flg]
  VINP_BMSWarn6_flg/1 -> Fault level 3 subsystem error/7(VINP_BMSWarn6_flg)
  VINP_BMSWarn8_flg/1 -> Fault level 4 subsystem error/6(VINP_BMSWarn8_flg)
  VINP_BMSWarn7_flg/1 -> Fault level 4 subsystem error/5(VINP_BMSWarn7_flg)
  [VDDM_C3BMS6LCCFS_flg] -> Fault level 4 subsystem error/4(VDDM_C3BMS6LCCFS_flg)
  [VDDM_C3BMS6LCCFS_flg] -> Fault level 3 subsystem error/4(VDDM_C3BMS6LCCFS_flg)
  [VDDM_MCUR1NoComCFS_flg] -> Fault level 3 subsystem error/6(VDDM_MCUR1NoComCFS_flg)
  [VDDM_MCUF1NoComCFS_flg] -> Fault level 3 subsystem error/5(VDDM_MCUF1NoComCFS_flg)
  [VDDM_MCUF1NoComCFS_flg] -> Fault level 2 subsystem error/6(VDDM_MCUF1NoComCFS_flg)
  [VDDM_MCUR1NoComCFS_flg] -> Fault level 2 subsystem error/7(VDDM_MCUR1NoComCFS_flg)
  VINP_BMSWarn4_flg/1 -> Fault level 2 subsystem error/8(VINP_BMSWarn4_flg)
  VINP_BMSWarn5_flg/1 -> Fault level 2 subsystem error/9(VINP_BMSWarn5_flg)
  [VDDM_MCUF1NoComCFS_flg] -> Fault level 1 subsystem error/6(VDDM_MCUF1NoComCFS_flg)
  [VDDM_MCUR1NoComCFS_flg] -> Fault level 1 subsystem error/7(VDDM_MCUR1NoComCFS_flg)
  VDDM_MCUF1NoComCFS_flg/1 -> [VDDM_MCUF1NoComCFS_flg]
  VDDM_MCUR1NoComCFS_flg/1 -> [VDDM_MCUR1NoComCFS_flg]
  [VDDM_C3BMS6LCCFS_flg] -> Fault level 2 subsystem error/4(VDDM_C3BMS6LCCFS_flg)
  [VDDM_C3BMS6LCCFS_flg] -> Fault level 1 subsystem error/4(VDDM_C3BMS6LCCFS_flg)
  VDDM_C3BMS6LCCFS_flg/1 -> [VDDM_C3BMS6LCCFS_flg]
  [task_time_s] -> Fault level 4 subsystem error/1(task_time_s)
  [VPMM_DrivetrainSelect_enum] -> Fault level 1 subsystem error/15(VPMM_DrivetrainSelect_enum)
  VPMM_DrivetrainSelect_enum/1 -> [VPMM_DrivetrainSelect_enum]
  [task_time_s] -> Fault level 3 subsystem error/1(task_time_s)
  [VINP_DCDCFaultSta_enum] -> Fault level 1 subsystem error/11(VINP_DCDCFaultSta_enum)
  [VINP_DCDCFaultSta_enum] -> Fault level 2 subsystem error/10(VINP_DCDCFaultSta_enum)
  VINP_DCDCFaultSta_enum/1 -> [VINP_DCDCFaultSta_enum]
  [task_time_s] -> Fault level 2 subsystem error/1(task_time_s)
  [task_time_s] -> Fault level 1 subsystem error/1(task_time_s)
  VPMM_PowerSta_enum/1 -> [VPMM_PowerSta_enum]
  VPMM_PwrStaSW_enum/1 -> [VPMM_PwrStaSW_enum]
  task_time_s/1 -> [task_time_s]
  [VPMM_PwrStaSW_enum] -> Fault level 1 subsystem error/3(VPMM_PwrStaSW_enum)
  [VPMM_PowerSta_enum] -> Fault level 1 subsystem error/2(VPMM_PowerSta_enum)
  [VPMM_PwrStaSW_enum] -> Fault level 2 subsystem error/3(VPMM_PwrStaSW_enum)
  [VPMM_PowerSta_enum] -> Fault level 2 subsystem error/2(VPMM_PowerSta_enum)
  [VPMM_PwrStaSW_enum] -> Fault level 3 subsystem error/3(VPMM_PwrStaSW_enum)
  [VPMM_PowerSta_enum] -> Fault level 3 subsystem error/2(VPMM_PowerSta_enum)
  [VPMM_PowerSta_enum] -> Fault level 4 subsystem error/2(VPMM_PowerSta_enum)
  [VPMM_PwrStaSW_enum] -> Fault level 4 subsystem error/3(VPMM_PwrStaSW_enum)

== system ddm/DDM/DDM/PMM/Key authentication failed ==
  note: Diagnostics and Fault Handling
  note: Release Condition During Failure Detection
  note: Fail Safe Operation After Failure Decision
  note: Test Detection Criteria
  note: Release Condition After Failure Decision
  note: Test Pass Criteria
  note: Fail Safe Operation During Failure Detection
  task_time_s : Inport
  VPMM_PowerSta_enum : Inport  Port=2
  VPMM_PwrStaSW_enum : Inport  Port=3
  VDDM_BrakeSW_enum : Inport  Port=4
  DTC_clear_request : Inport  Port=5
  VDKC_DKCAuthSta_enum : Inport  Port=6
  VINP_CANMsgValidDKC1_flg : Inport  Port=7
  VINP_CANMsgValidDKC2_flg : Inport  Port=8
  Constant1 : Constant  Value=ENUM_PWRSTASW_READY
  Constant11 : Constant  Value=KDDM_KeyAuthPassSW_flg
  Constant15 : Constant  Value=KDDM_KeyAuthCFSSW_flg
  Constant16 : Constant  Value=TRUE
  Constant19 : Constant  Value=ENUM_POWERSTA_OFF
  Constant{2,4,21,25,27} (5 alike) : Constant  Value=FALSE
  Constant20 : Constant  Value=KDDM_KeyAuthDFSSW_flg
  Constant24 : Constant  Value=TRUE
  Constant26 : Constant  Value=ENUM_PWRSTASW_READY
  Constant3 : Constant  Value=ENUM_BRKSW_ON
  Constant38 : Constant  Value=KDDM_KeyAuthDetTO_s
  Constant40 : Constant  Value=KDDM_KeyAuthDTC_cnt
  Constant43 : Constant  Value=KDDM_KeyAuthPassTO_s
  Constant44 : Constant  Value=KDDM_KeyAuthDetSW_flg
  Constant5 : Constant  Value=ENUM_BRKSW_ON
  Constant7 : Constant  Value=KDDM_KeyAuthPassTO_s
  Constant8 : Constant  Value=KDDM_KeyAuthDTC_cnt
  DTC_Couter : hcu_lib/Basic_Blocks/DTC_Couter
  DTC_Info : hcu_lib/Basic_Blocks/DTC_Info
  Data Type Conversion1 : DataTypeConversion  OutDataTypeStr=uint8
  Equal{,1..3,5} (5 alike) : RelationalOperator  Operator===  OutDataTypeStr=boolean  RndMeth=Simplest
  Equal4 : RelationalOperator  OutDataTypeStr=boolean  RndMeth=Simplest
  Logical Operator1 : Logic  Inputs=4  AllPortsSameDT=off  OutDataTypeStr=boolean
  Logical Operator12 : Logic  AllPortsSameDT=off  OutDataTypeStr=boolean
  Logical Operator15 : Logic  AllPortsSameDT=off  OutDataTypeStr=boolean
  Logical Operator18 : Logic  AllPortsSameDT=off  OutDataTypeStr=boolean
  Logical Operator19 : Logic  Inputs=3  AllPortsSameDT=off  OutDataTypeStr=boolean
  Logical Operator2 : Logic  Inputs=4  AllPortsSameDT=off  OutDataTypeStr=boolean
  Logical Operator3 : Logic  Operator=OR  Inputs=3  AllPortsSameDT=off  OutDataTypeStr=boolean
  Logical Operator4 : Logic  Operator=NOT  AllPortsSameDT=off  OutDataTypeStr=boolean
  Logical Operator5 : Logic  Operator=OR  AllPortsSameDT=off  OutDataTypeStr=boolean
  Logical Operator6 : Logic  Operator=NOT  AllPortsSameDT=off  OutDataTypeStr=boolean
  Logical Operator7 : Logic  Operator=OR  AllPortsSameDT=off  OutDataTypeStr=boolean
  Logical Operator8 : Logic  Operator=OR  AllPortsSameDT=off  OutDataTypeStr=boolean
  Relay : Relay  OnSwitchValue=ONE_INT  OffSwitchValue=ZERO_INT
  SR_Latch1 : Subsystem  mask(SR_Latch){}
      mask help: SR latch function.
  SR_Latch3 : hcu_lib/Basic_Blocks/SR_Latch
  SR_Latch4 : hcu_lib/Basic_Blocks/SR_Latch
  Switch{,1,4..6} (5 alike) : Switch  Criteria=u2 ~= 0
  Test Detection Criteria : hcu_lib/Basic_Blocks/Test Detection Criteria
  Timer1 : hcu_lib/Basic_Blocks/Timer
  VDDM_KeyAuthDTC_raw32 : Outport
  VDDM_EDriveSysErrKeyAuth_flg : Outport  Port=2
  wires:
  Logical Operator4/1 -> Logical Operator19/3
  Constant8/1 -> DTC_Couter/3
  [DTC_clear_request] -> Logical Operator3/3
  Logical Operator5/1 -> SR_Latch4/2
  [DTC_clear_request] -> Logical Operator5/2
  SR_Latch4/1 -> Logical Operator18/1
  Constant20/1 -> Logical Operator12/1
  SR_Latch3/1 -> Logical Operator12/2
  [VDDM_KeyAuthCFSRls_flg] -> Logical Operator5/1
  DTC_Couter/1 -> SR_Latch4/1
  [VDDM_KeyAuthDet_flg] -> Logical Operator19/1
  Logical Operator19/1 -> DTC_Couter/1
  Logical Operator12/1 -> [VDDM_KeyAuthDFS_flg]  "VDDM_KeyAuthDFS_flg"
  DTC_Couter/2 -> Data Type Conversion1/1
  Relay/1 -> SR_Latch3/1
  [VDDM_KeyAuthDTC_cnt] -> Relay/1
  Data Type Conversion1/1 -> [VDDM_KeyAuthDTC_cnt]  "VDDM_KeyAuthDTC_cnt"
  Constant44/1 -> Logical Operator19/2
  Logical Operator3/1 -> Logical Operator15/1
  [DTC_clear_request] -> Logical Operator4/1
  Constant15/1 -> Logical Operator18/2
  Logical Operator15/1 -> DTC_Couter/2
  [VDDM_KeyAuthPass_flg] -> Logical Operator3/1
  [VDDM_KeyAuthCFS_flg] -> Logical Operator7/1
  [VDDM_KeyAuthCFSRls_flg] -> Logical Operator3/2
  Constant11/1 -> Logical Operator15/2
  Logical Operator18/1 -> [VDDM_KeyAuthCFS_flg]  "VDDM_KeyAuthCFS_flg"
  [DTC_clear_request] -> Logical Operator7/2
  Logical Operator7/1 -> SR_Latch3/2
  [VDDM_xxx_flg] -> SR_Latch1/2(reset)
  Constant2/1 -> Switch6/1
  Switch5/1 -> Switch6/3, [VDDM_xxx_flg]
  Switch6/1 -> Test Detection Criteria/1
  [DTC_clear_request] -> Switch6/2
  [DTC_clear_request] -> DTC_Info/4
  Constant38/1 -> Test Detection Criteria/4
  [VDDM_KeyAuthDet_flg] -> DTC_Info/1
  DTC_Info/1 -> VDDM_KeyAuthDTC_raw32/1  "VDDM_KeyAuthDTC_raw32"
  [VDDM_KeyAuthCFS_flg] -> DTC_Info/3
  [VDDM_KeyAuthPass_flg] -> DTC_Info/2
  [task_time_s] -> Timer1/3
  [VDDM_EDriveSysErrKeyAuth_flg] -> VDDM_EDriveSysErrKeyAuth_flg/1
  DTC_clear_request/1 -> [DTC_clear_request]
  [VDKC_DKCAuthSta_enum] -> Switch5/1
  Constant3/1 -> Equal2/2
  [VDDM_BrakeSW_enum] -> Equal2/1
  Equal2/1 -> Logical Operator2/2
  [DTC_clear_request] -> Logical Operator8/2
  Equal5/1 -> Logical Operator8/1
  Constant7/1 -> Equal4/2
  Equal4/1 -> SR_Latch1/1(set)
  Constant25/1 -> Switch4/3
  Test Detection Criteria/1 -> [VDDM_KeyAuthDet_flg]  "VDDM_KeyAuthDet_flg"
  Constant21/1 -> Switch/3
  Switch4/1 -> [VDDM_KeyAuthCFSRls_flg]  "VDDM_KeyAuthCFSRls_flg"
  Logical Operator8/1 -> Switch4/2
  Constant19/1 -> Equal5/2
  Logical Operator2/1 -> Switch5/2
  Constant16/1 -> Switch/1
  [VPMM_PowerSta_enum] -> Equal5/1
  Switch/1 -> [VDDM_EDriveSysErrKeyAuth_flg]
  Switch1/1 -> Logical Operator6/1, Timer1/2
  Equal/1 -> Logical Operator2/1
  Constant24/1 -> Switch4/1
  Constant27/1 -> Switch5/3
  [VDDM_KeyAuthCFS_flg] -> Switch/2
  SR_Latch1/1(latched) -> [VDDM_KeyAuthPass_flg]  "VDDM_KeyAuthPass_flg"
  Logical Operator6/1 -> Timer1/1
  Constant26/1 -> Equal/2
  Constant43/1 -> Timer1/4
  Constant40/1 -> Test Detection Criteria/3
  [task_time_s] -> Test Detection Criteria/2
  [VPMM_PwrStaSW_enum] -> Equal/1
  Timer1/1 -> Equal4/1
  VDKC_DKCAuthSta_enum/1 -> [VDKC_DKCAuthSta_enum]
  VDDM_BrakeSW_enum/1 -> [VDDM_BrakeSW_enum]
  task_time_s/1 -> [task_time_s]
  VPMM_PwrStaSW_enum/1 -> [VPMM_PwrStaSW_enum]
  VPMM_PowerSta_enum/1 -> [VPMM_PowerSta_enum]
  VINP_CANMsgValidDKC1_flg/1 -> [VINP_CANMsgValidDKC1_flg]
  VINP_CANMsgValidDKC2_flg/1 -> [VINP_CANMsgValidDKC2_flg]
  [VINP_CANMsgValidDKC1_flg] -> Logical Operator2/3
  [VINP_CANMsgValidDKC2_flg] -> Logical Operator2/4
  Constant1/1 -> Equal1/2
  [VDDM_BrakeSW_enum] -> Equal3/1
  [VPMM_PwrStaSW_enum] -> Equal1/1
  Logical Operator1/1 -> Switch1/2
  Constant5/1 -> Equal3/2
  [VDKC_DKCAuthSta_enum] -> Switch1/1
  Equal3/1 -> Logical Operator1/2
  Constant4/1 -> Switch1/3
  [VINP_CANMsgValidDKC2_flg] -> Logical Operator1/4
  Equal1/1 -> Logical Operator1/1
  [VINP_CANMsgValidDKC1_flg] -> Logical Operator1/3

== system ddm/DDM/DDM/PMM/LV ==
  task_time_s : Inport
  VPMM_PwrStaSW_enum : Inport  Port=2
  VPMM_PowerSta_enum : Inport  Port=3
  VINP_LVBattDet12V_V : Inport  Port=4
  VINP_CANMsgValidBMS2_flg : Inport  Port=5
  DTC_clear_request : Inport  Port=6
  Initial LV battery voltage too low : Subsystem
  LV power supply voltage too high : Subsystem
  LV power supply voltage too low : Subsystem
  VDDM_IniLVLoDTC_raw32 : Outport
  VDDM_LVSupLoDTC_raw32 : Outport  Port=2
  VDDM_LVSupHiDTC_raw32 : Outport  Port=3
  wires:
  DTC_clear_request/1 -> [DTC_clear_request]
  LV power supply voltage too high/1(VDDM_LVSupHiDTC_raw32) -> VDDM_LVSupHiDTC_raw32/1
  [DTC_clear_request] -> LV power supply voltage too high/6(DTC_clear_request)
  [VINP_LVBattDet12V_V] -> LV power supply voltage too high/4(VINP_LVBattDet12V_V)
  [VPMM_PowerSta_enum] -> LV power supply voltage too high/2(VPMM_PowerSta_enum)
  [VINP_CANMsgValidBMS2_flg] -> LV power supply voltage too high/5(VINP_CANMsgValidBMS2_flg)
  [VPMM_PwrStaSW_enum] -> LV power supply voltage too high/3(VPMM_PwrStaSW_enum)
  [task_time_s] -> LV power supply voltage too high/1(task_time_s)
  [VINP_LVBattDet12V_V] -> LV power supply voltage too low/4(VINP_LVBattDet12V_V)
  [VINP_CANMsgValidBMS2_flg] -> LV power supply voltage too low/5(VINP_CANMsgValidBMS2_flg)
  LV power supply voltage too low/1(VDDM_LVSupLoDTC_raw32) -> VDDM_LVSupLoDTC_raw32/1
  [task_time_s] -> LV power supply voltage too low/1(task_time_s)
  [DTC_clear_request] -> LV power supply voltage too low/6(DTC_clear_request)
  [VPMM_PwrStaSW_enum] -> LV power supply voltage too low/3(VPMM_PwrStaSW_enum)
  [VPMM_PowerSta_enum] -> LV power supply voltage too low/2(VPMM_PowerSta_enum)
  Initial LV battery voltage too low/1(VDDM_IniLVLoDTC_raw32) -> VDDM_IniLVLoDTC_raw32/1
  [VPMM_PowerSta_enum] -> Initial LV battery voltage too low/2(VPMM_PowerSta_enum)
  [VPMM_PwrStaSW_enum] -> Initial LV battery voltage too low/3(VPMM_PwrStaSW_enum)
  [DTC_clear_request] -> Initial LV battery voltage too low/6(DTC_clear_request)
  [VINP_CANMsgValidBMS2_flg] -> Initial LV battery voltage too low/5(VINP_CANMsgValidBMS2_flg)
  [VINP_LVBattDet12V_V] -> Initial LV battery voltage too low/4(VINP_LVBattDet12V_V)
  [task_time_s] -> Initial LV battery voltage too low/1(task_time_s)
  VINP_CANMsgValidBMS2_flg/1 -> [VINP_CANMsgValidBMS2_flg]
  VINP_LVBattDet12V_V/1 -> [VINP_LVBattDet12V_V]
  task_time_s/1 -> [task_time_s]
  VPMM_PwrStaSW_enum/1 -> [VPMM_PwrStaSW_enum]
  VPMM_PowerSta_enum/1 -> [VPMM_PowerSta_enum]

== system ddm/DDM/DDM/PMM/SW failure ==
  task_time_s : Inport
  VPMM_PwrStaSW_enum : Inport  Port=2
  VPMM_PowerSta_enum : Inport  Port=3
  DTC_clear_request : Inport  Port=4
  VINP_DrStSW : Inport  Port=5
  VINP_FLAJARSW : Inport  Port=6
  VINP_FRAJARSW : Inport  Port=7
  VINP_RLAJARSW : Inport  Port=8
  VINP_RRAJARSW : Inport  Port=9
  VINP_HoodSW : Inport  Port=10
  VINP_TailgaSW : Inport  Port=11
  Driver seat switch failure : Subsystem
  FL Door switch failure : Subsystem
  FR Door switch failure : Subsystem
  Hood switch failure : Subsystem
  RL Door switch failure : Subsystem
  RR Door switch failure : Subsystem
  Tailgate switch failure : Subsystem
  VDDM_DrStSWDTC_raw32 : Outport
  VDDM_FLDoorSWDTC_raw32 : Outport  Port=2
  VDDM_RLDoorSWDTC_raw32 : Outport  Port=3
  VDDM_FRDoorSWDTC_raw32 : Outport  Port=4
  VDDM_RRDoorSWDTC_raw32 : Outport  Port=5
  VDDM_HoodSWDTC_raw32 : Outport  Port=6
  VDDM_TailgaSWDTC_raw32 : Outport  Port=7
  VDDM_DrSeatSta_enum : Outport  Port=8
  VDDM_VCUFLDoorSta_flg : Outport  Port=9
  VDDM_VCUFRDoorSta_flg : Outport  Port=10
  VDDM_VCURLDoorSta_flg : Outport  Port=11
  VDDM_VCURRDoorSta_flg : Outport  Port=12
  VDDM_VCUHoodSWSta_flg : Outport  Port=13
  VDDM_VCUTailgateSWSta_flg : Outport  Port=14
  wires:
  Tailgate switch failure/2(VDDM_VCUTailgateSWSta_flg) -> VDDM_VCUTailgateSWSta_flg/1
  Tailgate switch failure/1(VDDM_TailgaSWDTC_raw32) -> VDDM_TailgaSWDTC_raw32/1
  [VINP_TailgaSW] -> Tailgate switch failure/4(VINP_TailgaSW)
  [DTC_clear_request] -> Tailgate switch failure/5(DTC_clear_request)
  [VPMM_PwrStaSW_enum] -> Tailgate switch failure/3(VPMM_PwrStaSW_enum)
  [VPMM_PowerSta_enum] -> Tailgate switch failure/2(VPMM_PowerSta_enum)
  [task_time_s] -> Tailgate switch failure/1(task_time_s)
  Hood switch failure/2(VDDM_VCUHoodSWSta_flg) -> VDDM_VCUHoodSWSta_flg/1
  Hood switch failure/1(VDDM_HoodSWDTC_raw32) -> VDDM_HoodSWDTC_raw32/1
  [DTC_clear_request] -> Hood switch failure/5(DTC_clear_request)
  [VINP_HoodSW] -> Hood switch failure/4(VINP_HoodSW)
  VINP_TailgaSW/1 -> [VINP_TailgaSW]
  VINP_HoodSW/1 -> [VINP_HoodSW]
  [VPMM_PwrStaSW_enum] -> Hood switch failure/3(VPMM_PwrStaSW_enum)
  [VPMM_PowerSta_enum] -> Hood switch failure/2(VPMM_PowerSta_enum)
  [task_time_s] -> Hood switch failure/1(task_time_s)
  RR Door switch failure/2(VDDM_VCURRDoorSta_flg) -> VDDM_VCURRDoorSta_flg/1
  RR Door switch failure/1(VDDM_RRDoorSWDTC_raw32) -> VDDM_RRDoorSWDTC_raw32/1
  [DTC_clear_request] -> RR Door switch failure/5(DTC_clear_request)
  [VINP_RRAJARSW] -> RR Door switch failure/4(VINP_RRAJARSW)
  [VPMM_PwrStaSW_enum] -> RR Door switch failure/3(VPMM_PwrStaSW_enum)
  [VPMM_PowerSta_enum] -> RR Door switch failure/2(VPMM_PowerSta_enum)
  [task_time_s] -> RR Door switch failure/1(task_time_s)
  RL Door switch failure/2(VDDM_VCURLDoorSta_flg) -> VDDM_VCURLDoorSta_flg/1
  RL Door switch failure/1(VDDM_RLDoorSWDTC_raw32) -> VDDM_RLDoorSWDTC_raw32/1
  [DTC_clear_request] -> RL Door switch failure/5(DTC_clear_request)
  [VINP_RLAJARSW] -> RL Door switch failure/4(VINP_RLAJARSW)
  [task_time_s] -> RL Door switch failure/1(task_time_s)
  [VPMM_PowerSta_enum] -> RL Door switch failure/2(VPMM_PowerSta_enum)
  [VPMM_PwrStaSW_enum] -> RL Door switch failure/3(VPMM_PwrStaSW_enum)
  FR Door switch failure/2(VDDM_VCUFRDoorSta_flg) -> VDDM_VCUFRDoorSta_flg/1
  FR Door switch failure/1(VDDM_FRDoorSWDTC_raw32) -> VDDM_FRDoorSWDTC_raw32/1
  [DTC_clear_request] -> FR Door switch failure/5(DTC_clear_request)
  [VINP_FRAJARSW] -> FR Door switch failure/4(VINP_FRAJARSW)
  [VPMM_PwrStaSW_enum] -> FR Door switch failure/3(VPMM_PwrStaSW_enum)
  [VPMM_PowerSta_enum] -> FR Door switch failure/2(VPMM_PowerSta_enum)
  [task_time_s] -> FR Door switch failure/1(task_time_s)
  FL Door switch failure/2(VDDM_VCUFLDoorSta_flg) -> VDDM_VCUFLDoorSta_flg/1
  FL Door switch failure/1(VDDM_FLDoorSWDTC_raw32) -> VDDM_FLDoorSWDTC_raw32/1
  [DTC_clear_request] -> FL Door switch failure/5(DTC_clear_request)
  [VINP_FLAJARSW] -> FL Door switch failure/4(VINP_FLAJARSW)
  [VPMM_PwrStaSW_enum] -> FL Door switch failure/3(VPMM_PwrStaSW_enum)
  [VPMM_PowerSta_enum] -> FL Door switch failure/2(VPMM_PowerSta_enum)
  [task_time_s] -> FL Door switch failure/1(task_time_s)
  VINP_RRAJARSW/1 -> [VINP_RRAJARSW]
  VINP_RLAJARSW/1 -> [VINP_RLAJARSW]
  VINP_FRAJARSW/1 -> [VINP_FRAJARSW]
  VINP_FLAJARSW/1 -> [VINP_FLAJARSW]
  Driver seat switch failure/2(VDDM_DrSeatSta_enum) -> VDDM_DrSeatSta_enum/1
  DTC_clear_request/1 -> [DTC_clear_request]
  VPMM_PowerSta_enum/1 -> [VPMM_PowerSta_enum]
  VPMM_PwrStaSW_enum/1 -> [VPMM_PwrStaSW_enum]
  task_time_s/1 -> [task_time_s]
  VINP_DrStSW/1 -> [VINP_DrStSW]
  [task_time_s] -> Driver seat switch failure/1(task_time_s)
  [VINP_DrStSW] -> Driver seat switch failure/4(VINP_DrStSW)
  [DTC_clear_request] -> Driver seat switch failure/5(DTC_clear_request)
  [VPMM_PwrStaSW_enum] -> Driver seat switch failure/3(VPMM_PwrStaSW_enum)
  [VPMM_PowerSta_enum] -> Driver seat switch failure/2(VPMM_PowerSta_enum)
  Driver seat switch failure/1(VDDM_DrStSWDTC_raw32) -> VDDM_DrStSWDTC_raw32/1
